simulink model "mutirotor"  (R2023a)
settings: Solver=FixedStepAuto  StartTime=0.0  StopTime=50  FixedStep=framePeriod_s  RelTol=1e-3
undefined symbols (not defined in the file): Aircraft, DiscIntNeverNeededParam, framePeriod_s, frameRate_hz, magnitude
libraries: simulink x39, slpidlib x14, dspmathops x1
(part 1 of 4)
settings Model: Creator=brian  LastModifiedBy=tuan
settings SolverCC: AlgebraicLoopSolver=TrustRegion
settings OptimizationCC: DefaultParameterBehavior=Inlined  GainParamInheritBuiltInType=on  UseFloatMulNetSlope=on  DefaultUnderspecifiedDataType=single  EnhancedBackFolding=on  BooleansAsBitfields=on  PassReuseOutputArgsAs=Individual arguments  StateBitsets=on  DataBitsets=on  ActiveStateOutputEnumStorageType=uint16  ZeroExternalMemoryAtStartup=off  ZeroInternalMemoryAtStartup=off  EfficientFloat2IntCast=on  LifeSpan=inf  DifferentSizesBufferReuse=on  OptimizationPriority=RAM  OptimizationCustomize=off  EfficientTunableParamExpr=on
settings DebuggingCC: ParameterPrecisionLossMsg=none  ParameterTunabilityLossMsg=error  UnconnectedInputMsg=warning  UnconnectedOutputMsg=warning  UnconnectedLineMsg=warning  BusObjectLabelMismatch=error  RootOutportRequireBusObject=error  NonBusSignalsTreatedAsBus=error  SFInvalidInputDataAccessInChartInitDiag=error  SFTransitionOutsideNaturalParentDiag=error  SFUnreachableExecutionPathDiag=error  SFUndirectedBroadcastEventsDiag=error
settings HardwareCC: ProdBitPerPointer=32  ProdBitPerSizeT=32  ProdBitPerPtrDiffT=32  ProdLargestAtomicInteger=Long  ProdLargestAtomicFloat=Double  ProdWordSize=32  ProdHWDeviceType=NXP->Cortex-M4  TargetLargestAtomicInteger=Long  TargetLargestAtomicFloat=Double  TargetLongLongMode=on  TargetIntDivRoundTo=Zero  TargetEndianess=LittleEndian  TargetHWDeviceType=NXP->Cortex-M4  ProdEqTarget=off
settings ModelReferenceCC: EnableRefExpFcnMdlSchedulingChecks=on  ModelReferenceNumInstancesAllowed=Single
settings SFSimCC: SimParseCustomCode=off  SimGenImportedTypeDefs=on  MATLABDynamicMemAlloc=off  SimTargetLang=C++
settings SFSimCC: SimUserIncludeDirs=|
  | ../../flight_code/include
  | ../../../ua_spaaro_extra/imu/include
  | ../../../ua_spaaro_extra/gnss/include
  | ../../../ua_spaaro_extra/pres/include
  | ../../../ua_spaaro_extra/sbus/include
  | ../../../ua_spaaro_extra/global_defs/include
settings SFSimCC: SimUserDefines=|
  | SIL
  | __FMU_R_MINI_V1__
settings RTWCC: Description=Embedded Coder  SystemTargetFile=ert.tlc  GenCodeOnly=on  TemplateMakefile=ert_default_tmf  GenerateReport=on  RTWVerbose=off  RTWUseSimCustomCode=on  Toolchain=GNU gcc/g++ | gmake (64-bit Linux)  BuildConfiguration=Specify  IncludeHyperlinkInReport=on  LaunchReport=on  TargetLang=C++  GenerateTraceInfo=on  GenerateTraceReport=on  GenerateTraceReportSl=on  GenerateTraceReportSf=on  GenerateTraceReportEml=on  GenerateCodeReplacementReport=on  DLArmComputeVersion=19.05
settings RTWCC: CustomInclude=|
  | ../../flight_code/include
  | ../../../ua_spaaro_extra/imu/include
  | ../../../ua_spaaro_extra/gnss/include
  | ../../../ua_spaaro_extra/pres/include
  | ../../../ua_spaaro_extra/sbus/include
  | ../../../ua_spaaro_extra/global_defs/include
settings RTWCC: CustomDefine=|
  | SIL
  | __FMU_R_MINI_V1__
settings CodeAppCC: ForceParamTrailComments=on  IgnoreCustomStorageClasses=off  OperatorAnnotations=on  SimulinkDataObjDesc=on  SFDataObjDesc=on  MATLABFcnDesc=on  CustomSymbolStrGlobalVar=rt$N$M  CustomSymbolStrType=$N$M  CustomSymbolStrFcn=$N$M$F  CustomSymbolStrMacro=$N$M  InsertBlockDesc=on  StateflowObjectComments=on  MATLABSourceComments=on  EnableCustomComments=on  InternalIdentifier=Classic  InlinedPrmAccess=Macros  ReqsInCode=on
settings ERTTargetCC: TargetLangStandard=C++03 (ISO)  GenerateFullHeader=off  IncludeMdlTerminateFcn=off  CombineSignalStateStructs=on  SuppressErrorStatus=on  SupportAbsoluteTime=off  CodeInterfacePackaging=C++ class  SupportNonFinite=off  SupportComplex=off  ParenthesesLevel=Standards  CastingMode=Standards  ERTHeaderFileRootName=autocode$E  ERTSourceFileRootName=autocode$E  InlinedParameterPlacement=NonHierarchical  RootIOFormat=Structure reference  ERTCustomFileTemplate=example_file_process.tlc  ERTFilePackagingFormat=Compact  PreserveExpressionOrder=on  PreserveIfCondition=on  ConvertIfToSwitch=off  EnableSignedLeftShifts=off  EnableSignedRightShifts=off  IndentSize=4

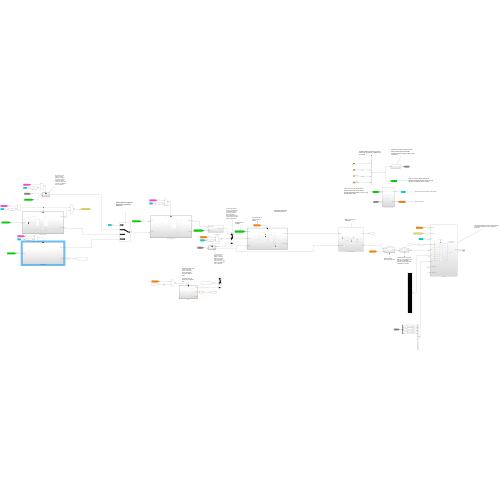
[thumbnail: Simulink's stored preview of the top-level diagram]
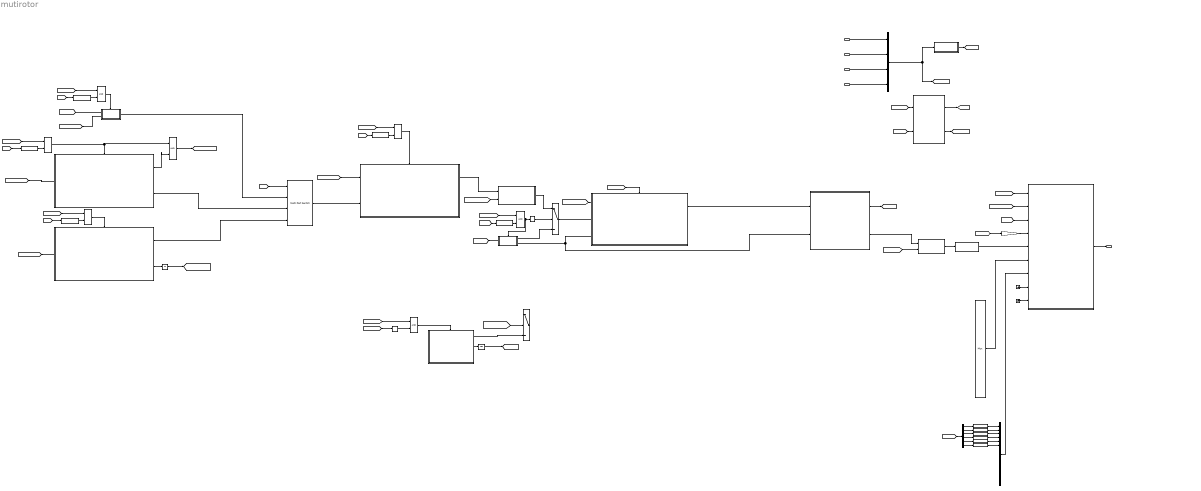
== system mutirotor ==
  note: Combine different data structures or buses into one bus for convenient of accessing
  note: Extract the inceptor channel to form some common pilot commands. Combine them to a single "cmd" bus for convenient
  note: This is a "Go To" tag. It acts like a wireless connection in the model. This is used for cleanliness of the model
  note: This is a "From" tag. It acts like a wireless connection in the model, accessing the data from the "Go To" tag with the same name
  note: This block should be used in all VMS model to format all data to the correct type for autocode.
  note: Convert motor commands from 0 to 1 into PWM value from 1100 to 1900 (or whatever range supported by the ESC or servos)
  note: System to stop motor if E-Stop is hit
  note: Motor mixing and saturation
  note: Mode signal for logging and flight_mode switching
  note: Motor arming signal
  note: ANGLE AND ANGULAR RATE CONTROLLER
  note: This ensure calc is only done when needed
  note: All data used for feedback
  note: For cascaded control scheme, controllers has a commond interface. This block switch the input of the angle control between pilot or a higher order controller based on flight mode
  note: For pilot input, the sticks can mean different command depending on flight mode. This block conver the same stick command to different state commands
  note: Autonomous Take Off mode. Just ramp motor to 70% and send it. Work well enough for MALT in cage.
      |
      | Need more testing before used anywhere else
  note: Select different input for the velocity controller interface
  note: For pilot input, the sticks can mean different command depending on flight mode. This block conver the same stick command to different state commands
  System Data : Inport  OutDataTypeStr=Bus: SysData  SampleTime=framePeriod_s  BusOutputAsStruct=on
  Sensor Data : Inport  Port=2  OutDataTypeStr=Bus: SensorData  SampleTime=framePeriod_s  BusOutputAsStruct=on
  StateEstData : Inport  Port=3  OutDataTypeStr=Bus: StateEstData  SampleTime=framePeriod_s  BusOutputAsStruct=on
  Telemetry Data : Inport  Port=4  OutDataTypeStr=Bus: TelemData  SampleTime=framePeriod_s  BusOutputAsStruct=on
  AND : Logic  IconShape=distinctive  AllPortsSameDT=off  OutDataTypeStr=boolean
  ANGLE CONTROLLER1 : Subsystem
  BODY_ACC_TO_ANGLE_CONVERSION : Subsystem
  Bus Creator1 : BusCreator  Inputs=4
  Bus Selector4 : BusSelector  OutputSignals=throttle,pitch,roll,yaw,e-stop,mode
  Cast To Single{,1..5} (6 alike) : DataTypeConversion  OutDataTypeStr=int16  SaturateOnIntegerOverflow=off  RndMeth=Floor
  Gain : Gain  Gain=100
  Ground : Ground
  Ground1 : Ground
  LAND CONTROLLER : Subsystem
  Motor Mixing Algorithm : Subsystem
  Multiport Switch : MultiPortSwitch  SaturateOnIntegerOverflow=off  InputSameDT=off
  Mux : Mux  Inputs=24
  Mux1 : Mux  Inputs=16
  NOT : Logic  Operator=NOT  IconShape=distinctive  AllPortsSameDT=off  OutDataTypeStr=boolean
  NOT1 : Logic  Operator=NOT  IconShape=distinctive  AllPortsSameDT=off  OutDataTypeStr=boolean
  POS_HOLD CONTROLLER : Subsystem
  POS_HOLD_input_conversion : Subsystem
  Stab_input_conversion : Subsystem
  Switch : Switch  Criteria=u2 > Threshold  Threshold=0.5  SaturateOnIntegerOverflow=off  InputSameDT=off
  Switch1 : Switch  Criteria=u2 > Threshold  Threshold=0.5  SaturateOnIntegerOverflow=off  InputSameDT=off
  TAKE-OFF : Subsystem
  To VMS Data1 : Subsystem
  Unit Delay : UnitDelay  SampleTime=framePeriod_s  HasFrameUpgradeWarning=on
  Unit Delay1 : UnitDelay  SampleTime=framePeriod_s  HasFrameUpgradeWarning=on
  WAYPOINT CONTROLLER : Subsystem
  cmd to raw pwm : Subsystem
  command selection : Subsystem
  compare_to_pos_hold : simulink/Logic and Bit Operations/Compare To Constant  relop=>=  const=1  OutDataTypeStr=boolean
  compare_to_stab : simulink/Logic and Bit Operations/Compare To Constant  relop===  const=0  OutDataTypeStr=boolean
  compare_to_stab1 : simulink/Logic and Bit Operations/Compare To Constant  relop===  const=1  OutDataTypeStr=boolean
  compare_to_wp : simulink/Logic and Bit Operations/Compare To Constant  relop===  const=2  OutDataTypeStr=boolean
  compare_to_wp1 : simulink/Logic and Bit Operations/Compare To Constant  relop=>=  const=3  OutDataTypeStr=boolean
  determine arm and mode selection1 : Subsystem
  emergency_stop_system : Subsystem
  motor_armed AND mode_{0..5} (6 alike) : Logic  IconShape=distinctive  AllPortsSameDT=off  OutDataTypeStr=boolean
  VmsData : Outport  OutDataTypeStr=Bus: VmsData  SampleTime=framePeriod_s  BusOutputAsStruct=on
  wires:
  To VMS Data1/1(VmsData) -> VmsData/1  "VmsData"
  [Mode] -> To VMS Data1/3(Mode in)
  [arm_state] -> To VMS Data1/1(motors_enabled)
  [throttle] -> Gain/1
  command selection/1(cmd) -> [cmd]
  Bus Creator1/1 -> command selection/1(InBus), [sys_input]
  Motor Mixing Algorithm/2(PWM) -> emergency_stop_system/1(input_signal)
  cmd to raw pwm/1(PwmCmd) -> To VMS Data1/5(PWM In)  "PwmCmd"
  emergency_stop_system/1(pwm_cmd) -> cmd to raw pwm/1(pwm_cmd)
  Mux/1 -> To VMS Data1/6(Aux)
  [arm_state] -> emergency_stop_system/2(arm)
  compare_to_stab/1 -> motor_armed AND mode_0/2
  [cmd] -> Stab_input_conversion/1(cmd)
  [sys_input] -> ANGLE CONTROLLER1/1(Sys_input)
  [arm_state] -> motor_armed AND mode_0/1
  motor_armed AND mode_0/1 -> NOT/1, Stab_input_conversion/Enable
  [Mode] -> compare_to_stab/1
  ANGLE CONTROLLER1/1(Command out) -> Motor Mixing Algorithm/1(MMA Bus)
  compare_to_pos_hold/1 -> motor_armed AND mode_1/2
  motor_armed AND mode_5/1 -> POS_HOLD_input_conversion/Enable
  [cmd] -> POS_HOLD_input_conversion/1(cmd)
  [Mode] -> compare_to_pos_hold/1
  [arm_state] -> motor_armed AND mode_1/1
  [arm_state] -> motor_armed AND mode_5/1
  [Mode] -> compare_to_stab1/1
  motor_armed AND mode_1/1 -> POS_HOLD CONTROLLER/Enable
  compare_to_stab1/1 -> motor_armed AND mode_5/2
  System Data/1 -> Bus Creator1/1  "Sys Data"
  Sensor Data/1 -> Bus Creator1/2  "Sensor Data"
  StateEstData/1 -> Bus Creator1/3  "StateEstData"
  [sys_input] -> POS_HOLD CONTROLLER/1(Sys_input)
  AND/1 -> [waypoint_reached]
  motor_armed AND mode_2/1 -> WAYPOINT CONTROLLER/Enable, AND/1
  [arm_state] -> motor_armed AND mode_2/1
  [Mode] -> compare_to_wp/1
  compare_to_wp/1 -> motor_armed AND mode_2/2
  Multiport Switch/1 -> POS_HOLD CONTROLLER/2(Cmd_input)
  [sys_input] -> WAYPOINT CONTROLLER/1(Sys_input)
  WAYPOINT CONTROLLER/1(wp_reached) -> AND/2
  [cmd] -> Bus Selector4/1
  Bus Selector4/1 -> Cast To Single/1  "<throttle>"
  Bus Selector4/2 -> Cast To Single1/1  "<pitch>"
  Bus Selector4/3 -> Cast To Single2/1  "<roll>"
  Bus Selector4/4 -> Cast To Single3/1  "<yaw>"
  Bus Selector4/5 -> Cast To Single4/1  "<e-stop>"
  Bus Selector4/6 -> Cast To Single5/1  "<mode>"
  Cast To Single/1 -> Mux1/1
  Cast To Single1/1 -> Mux1/2
  Cast To Single2/1 -> Mux1/3
  Cast To Single3/1 -> Mux1/4
  Cast To Single4/1 -> Mux1/5
  Cast To Single5/1 -> Mux1/6
  Telemetry Data/1 -> Bus Creator1/4  "Telemetry Data"
  [sys_input] -> BODY_ACC_TO_ANGLE_CONVERSION/2(SysData)
  Switch/1 -> ANGLE CONTROLLER1/2(Cmd_input)
  Motor Mixing Algorithm/1(throttle) -> [throttle]
  NOT/1 -> Switch/2
  POS_HOLD CONTROLLER/1(Command out) -> BODY_ACC_TO_ANGLE_CONVERSION/1(Outer loop command)
  BODY_ACC_TO_ANGLE_CONVERSION/1(Inner loop command) -> Switch/1
  [sys_input] -> POS_HOLD_input_conversion/2(Sys)
  POS_HOLD_input_conversion/1(angle_ctrl_input) -> Multiport Switch/2
  WAYPOINT CONTROLLER/2(wp_command) -> Multiport Switch/3
  [arm_state] -> motor_armed AND mode_3/1
  compare_to_wp1/1 -> motor_armed AND mode_3/2
  [Mode] -> compare_to_wp1/1
  motor_armed AND mode_3/1 -> LAND CONTROLLER/Enable
  [sys_input] -> LAND CONTROLLER/1(Sys_input)
  LAND CONTROLLER/2(disarm_cc) -> Unit Delay/1
  [Mode] -> Multiport Switch/1
  LAND CONTROLLER/1(land_command) -> Multiport Switch/4
  [waypoint_reached] -> To VMS Data1/2(waypoint_reached)
  Unit Delay/1 -> [LAND_DISARM]
  TAKE-OFF/2(taken_off) -> Unit Delay1/1
  Unit Delay1/1 -> [TAKEN_OFF]
  [TAKEN_OFF] -> NOT1/1
  [arm_state] -> motor_armed AND mode_4/1
  motor_armed AND mode_4/1 -> TAKE-OFF/Enable
  NOT1/1 -> motor_armed AND mode_4/2
  [TAKEN_OFF] -> Switch1/2
  [arm_state] -> ANGLE CONTROLLER1/Enable
  TAKE-OFF/1(take_off) -> Switch1/3
  Gain/1 -> To VMS Data1/4(throttle_cmd_prcnt)
  Mux1/1 -> To VMS Data1/7(SBUS in)
  Ground/1 -> To VMS Data1/8(flight_time_remaining_s)
  Ground1/1 -> To VMS Data1/9(power_remaining_prcnt)
  [sys_input] -> determine arm and mode selection1/1(sys_input)
  determine arm and mode selection1/2(arm_state) -> [arm_state]
  determine arm and mode selection1/1(mode) -> [Mode]
  [cmd] -> determine arm and mode selection1/2(Cmd)
  Stab_input_conversion/1(angle_ctrl_input) -> Switch/3
  Stab_input_conversion/2(low_throttle) -> ANGLE CONTROLLER1/3(low_thottle), Motor Mixing Algorithm/2(low_throttle_flag)

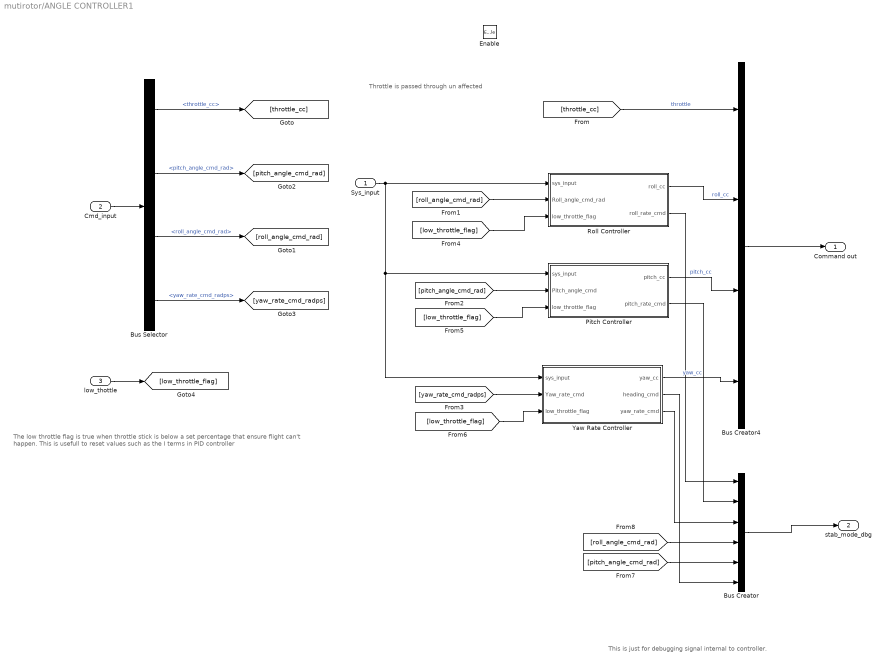
== system mutirotor/ANGLE CONTROLLER1 ==
  note: Throttle is passed through un affected
  note: The low throttle flag is true when throttle stick is below a set percentage that ensure flight can't happen. This is usefull to reset values such as the I terms in PID controller
  note: This is just for debugging signal internal to controller.
  Sys_input : Inport
  Cmd_input : Inport  Port=2
  low_thottle : Inport  Port=3
  Enable : EnablePort
  Bus Creator : BusCreator  Inputs=6
  Bus Creator4 : BusCreator  Inputs=4
  Bus Selector : BusSelector  OutputSignals=throttle_cc,pitch_angle_cmd_rad,roll_angle_cmd_rad,yaw_rate_cmd_radps
  Pitch Controller : Subsystem
  Roll Controller : Subsystem
  Yaw Rate Controller : Subsystem
  Command out : Outport
  stab_mode_dbg : Outport  Port=2
  wires:
  Bus Creator4/1 -> Command out/1
  Cmd_input/1 -> Bus Selector/1
  Yaw Rate Controller/1(yaw_cc) -> Bus Creator4/4  "yaw_cc"
  Pitch Controller/1(pitch_cc) -> Bus Creator4/3  "pitch_cc"
  Roll Controller/1(roll_cc) -> Bus Creator4/2  "roll_cc"
  Sys_input/1 -> Yaw Rate Controller/1(sys_input), Pitch Controller/1(sys_input), Roll Controller/1(sys_input)
  Bus Selector/1 -> [throttle_cc]  "<throttle_cc>"
  Bus Selector/4 -> [yaw_rate_cmd_radps]  "<yaw_rate_cmd_radps>"
  Bus Selector/2 -> [pitch_angle_cmd_rad]  "<pitch_angle_cmd_rad>"
  Bus Selector/3 -> [roll_angle_cmd_rad]  "<roll_angle_cmd_rad>"
  [throttle_cc] -> Bus Creator4/1  "throttle"
  [roll_angle_cmd_rad] -> Roll Controller/2(Roll_angle_cmd_rad)
  [pitch_angle_cmd_rad] -> Pitch Controller/2(Pitch_angle_cmd)
  [yaw_rate_cmd_radps] -> Yaw Rate Controller/2(Yaw_rate_cmd)
  low_thottle/1 -> [low_throttle_flag]
  [low_throttle_flag] -> Roll Controller/3(low_throttle_flag)
  [low_throttle_flag] -> Pitch Controller/3(low_throttle_flag)
  [low_throttle_flag] -> Yaw Rate Controller/3(low_throttle_flag)
  Roll Controller/2(roll_rate_cmd) -> Bus Creator/1
  Pitch Controller/2(pitch_rate_cmd) -> Bus Creator/2
  Bus Creator/1 -> stab_mode_dbg/1
  [roll_angle_cmd_rad] -> Bus Creator/4
  [pitch_angle_cmd_rad] -> Bus Creator/5
  Yaw Rate Controller/2(heading_cmd) -> Bus Creator/6
  Yaw Rate Controller/3(yaw_rate_cmd) -> Bus Creator/3

== system mutirotor/BODY_ACC_TO_ANGLE_CONVERSION ==
  note: The input here is the acceleration command in the earth frame in mps^2
  note: g is added to also compensate for gravity
  note: 10 deg tilt limit is pre computed
  note: Convert it to g
  note: Yaw rate command is unaffected
  note: Limit the thrust to match achivable thrust
      |
      | Prioritize vertical axis (0 lateral accel if needed)
  note: Limit max tilt of the thrust vector. Essential set a limit for tilt while ensureing the vertical accel is unchanged
  note: Conversion between thrust vector magnitude to throttle command
      |
      | The gain needs to be tunable
  note: Calculated the needed pitch and roll so that the aircraft thrust vector point in the direction of the commanded earth frame accel vector
      |
      | In this implementation, gimbal lock and inverted flight will cause problem.
      |
      | Better to implement quartenion based conversion and inner loop
  note: Construct a bus to match the inner controller interface
  Outer loop command : Inport
  SysData : Inport  Port=2
  " tilt_limiter" : MATLAB Function  TreatAsAtomicUnit=on
  Bus Creator : BusCreator  Inputs=4
  Bus Selector : BusSelector  OutputSignals=acc_x_cmd,acc_y_cmd,acc_z_cmd,yaw_rate_cmd_radps
  Bus Selector1 : BusSelector  OutputSignals=StateEstData.bfs_ins.heading_rad
  Constant : Constant  Value=Aircraft.Control.max_g_thr  OutDataTypeStr=single
  Constant1 : Constant  Value=Aircraft.Control.est_hover_thr  OutDataTypeStr=single
  Constant2 : Constant  Value=Aircraft.Control.max_g_thr  OutDataTypeStr=single
  Constant3 : Constant  Value=10  OutDataTypeStr=single
  Mux : Mux  Inputs=3
  Sum : Sum  Inputs=|+-
  calc_body_throttle : MATLAB Function  TreatAsAtomicUnit=on
  g : Constant  OutDataTypeStr=single
  normalize by g1 : Gain  Gain=1/9.81
  normalize by g2 : Gain  Gain=1/9.81
  normalize by g3 : Gain  Gain=1/9.81
  thrust_limit : MATLAB Function  TreatAsAtomicUnit=on
  tilt_command_calculation : MATLAB Function  TreatAsAtomicUnit=on
  Inner loop command : Outport
  wires:
  Constant/1 -> thrust_limit/2(max_thrust)
  Mux/1 -> thrust_limit/1(thrust_vector_raw)
  Outer loop command/1 -> Bus Selector/1
  Bus Selector/1 -> normalize by g1/1  "<acc_x_cmd>"
  Bus Selector/2 -> normalize by g2/1  "<acc_y_cmd>"
  Bus Creator/1 -> Inner loop command/1  "angle_ctrl_input"
  Bus Selector/4 -> Bus Creator/4  "<yaw_rate_cmd_radps>"
  SysData/1 -> Bus Selector1/1
  Bus Selector1/1 -> tilt_command_calculation/2(psi_rad)  "<heading_rad>"
  Bus Selector/3 -> normalize by g3/1  "<acc_z_cmd>"
  g/1 -> Sum/2
  normalize by g3/1 -> Sum/1
  normalize by g1/1 -> Mux/1
  normalize by g2/1 -> Mux/2
  Sum/1 -> Mux/3
  thrust_limit/1(limited_vector) -> " tilt_limiter"/1(thrust_vector_raw)
  tilt_command_calculation/1(phi_rad) -> Bus Creator/3  "roll_angle_cmd_rad"
  tilt_command_calculation/2(theta_rad) -> Bus Creator/2  "pitch_angle_cmd_rad"
  calc_body_throttle/1(throttle) -> Bus Creator/1  "throttle_cc"
  " tilt_limiter"/1(limited_vector) -> calc_body_throttle/1(raw_thrust_vector), tilt_command_calculation/1(thrust_vector_ned)
  Constant1/1 -> calc_body_throttle/2(hover_thr)
  Constant2/1 -> calc_body_throttle/3(max_g_thrust)
  Constant3/1 -> calc_body_throttle/4(gain)

== system mutirotor/LAND CONTROLLER ==
  note: LAND CONTROLLER IS EXPLAINED IN README
  Sys_input : Inport
  Enable : EnablePort  StatesWhenEnabling=reset  ShowOutputPort=on
  Bus Creator4 : BusCreator  Inputs=4
  Bus Selector : BusSelector  OutputSignals=Sensor Data.ext_gnss1.alt_wgs84_m
  Compare To Constant : simulink/Logic and Bit Operations/Compare To Constant  relop=<=  const=0.15  OutDataTypeStr=boolean
  Constant : Constant  Value=0  OutDataTypeStr=single
  Constant1 : Constant  Value=0  OutDataTypeStr=single
  Constant2 : Constant  Value=0  OutDataTypeStr=single
  Constant3 : Constant  Value=Aircraft.Control.v_z_max  OutDataTypeStr=single
  Enabled Subsystem : Subsystem  TreatAsAtomicUnit=on
  OR : Logic  Operator=OR  IconShape=distinctive  AllPortsSameDT=off  OutDataTypeStr=boolean
  land_command : Outport
  disarm_cc : Outport  Port=2
  wires:
  Bus Creator4/1 -> land_command/1
  Constant1/1 -> Bus Creator4/3  "ve_y_cmd_mps"
  Constant2/1 -> Bus Creator4/4  "yaw_rate_cmd_radps"
  Constant/1 -> Bus Creator4/2  "ve_x_cmd_mps"
  Constant3/1 -> Bus Creator4/1  "ve_z_cmd_mps"
  Sys_input/1 -> Bus Selector/1
  Bus Selector/1 -> Compare To Constant/1  "<alt_wgs84_m>"
  Compare To Constant/1 -> OR/1
  OR/1 -> disarm_cc/1
  Enabled Subsystem/1(LAND_MODE_TIMER) -> OR/2
  Enable/1 -> [LAND_ENABLED]
  [LAND_ENABLED] -> Enabled Subsystem/Enable

== system mutirotor/Motor Mixing Algorithm ==
  note: High level command multiply by mixing matrix
  note: Saturate minimum throttle command
  note: Extra precaution to ensure low throttle. Essentially any throttle below ~30% is no throttle at all
  note: High level commands
  MMA Bus : Inport
  low_throttle_flag : Inport  Port=2
  Bus Selector : BusSelector  OutputSignals=throttle,roll_cc,pitch_cc,yaw_cc
  Constant : Constant  OutDataTypeStr=single
  Constant1 : Constant  Value=Aircraft.Control.motor_spin_min  OutDataTypeStr=single
  Constant2 : Constant  Value=[0 0 0 0 0 0 0 0]  OutDataTypeStr=single
  Motor Mix : Constant  Value=Aircraft.Motor.mix  OutDataTypeStr=single
  Multiply : Product  Inputs=**  Multiplication=Matrix(*)  OutDataTypeStr=single
  Mux : Mux
  Reshape : Reshape  OutputDimensionality=Row vector (2-D)
  Saturation Dynamic : simulink/Discontinuities/Saturation Dynamic  OutMin=[]  OutMax=[]  OutDataTypeStr=Inherit: Same as second input  OutDataType=fixdt(1, 16)  OutScaling=2^-10  DoSatur=off
  Switch : Switch  Criteria=u2 > Threshold  SaturateOnIntegerOverflow=off  InputSameDT=off
  Transpose : Math  Operator=transpose
  throttle : Outport
  PWM : Outport  Port=2
  wires:
  Mux/1 -> Reshape/1
  Reshape/1 -> Multiply/1
  Motor Mix/1 -> Transpose/1
  MMA Bus/1 -> Bus Selector/1
  Bus Selector/1 -> Mux/1, throttle/1  "<throttle>"
  Transpose/1 -> Multiply/2
  Saturation Dynamic/1 -> PWM/1
  Constant/1 -> Saturation Dynamic/1
  Constant1/1 -> Saturation Dynamic/3
  Bus Selector/2 -> Mux/2  "<roll_cc>"
  Bus Selector/3 -> Mux/3  "<pitch_cc>"
  Bus Selector/4 -> Mux/4  "<yaw_cc>"
  Switch/1 -> Saturation Dynamic/2
  low_throttle_flag/1 -> Switch/2
  Multiply/1 -> Switch/3  "Command"
  Constant2/1 -> Switch/1

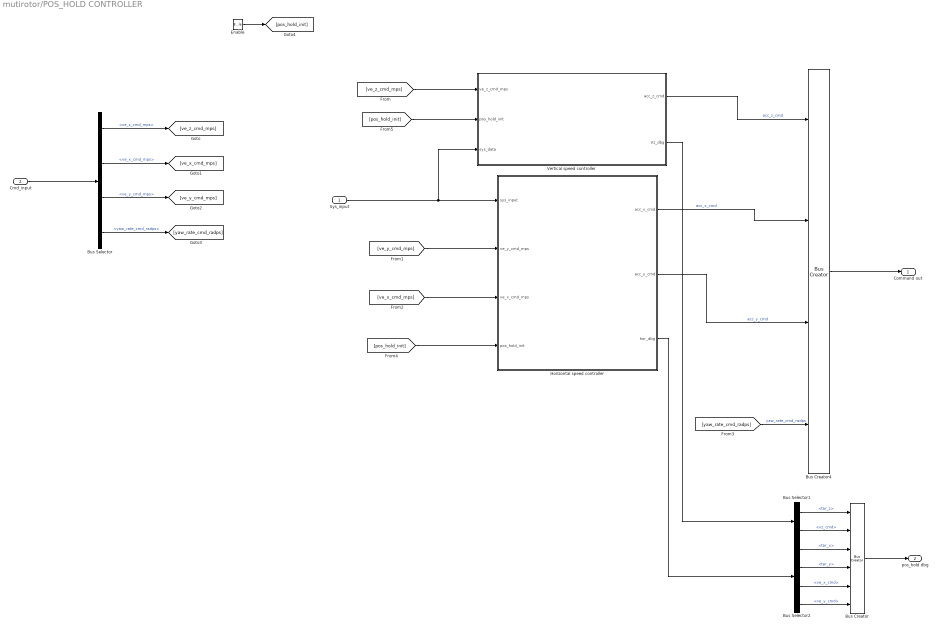
== system mutirotor/POS_HOLD CONTROLLER ==
  Sys_input : Inport
  Cmd_input : Inport  Port=2
  Enable : EnablePort  StatesWhenEnabling=reset  PropagateVarSize=During execution  ShowOutputPort=on
  Bus Creator : BusCreator  Inputs=6
  Bus Creator4 : BusCreator  Inputs=4
  Bus Selector : BusSelector  OutputSignals=ve_z_cmd_mps,ve_x_cmd_mps,ve_y_cmd_mps,yaw_rate_cmd_radps
  Bus Selector1 : BusSelector  OutputSignals=tar_z,vz_cmd
  Bus Selector2 : BusSelector  OutputSignals=tar_x,tar_y,ve_x_cmd,ve_y_cmd
  Horizontal speed controller : Subsystem
  Vertical speed controller : Subsystem
  Command out : Outport
  pos_hold dbg : Outport  Port=2
  wires:
  Bus Creator4/1 -> Command out/1
  Bus Selector/1 -> [ve_z_cmd_mps]  "<ve_z_cmd_mps>"
  Bus Selector/2 -> [ve_x_cmd_mps]  "<ve_x_cmd_mps>"
  Bus Selector/3 -> [ve_y_cmd_mps]  "<ve_y_cmd_mps>"
  Bus Selector/4 -> [yaw_rate_cmd_radps]  "<yaw_rate_cmd_radps>"
  [yaw_rate_cmd_radps] -> Bus Creator4/4  "yaw_rate_cmd_radps"
  Cmd_input/1 -> Bus Selector/1
  Enable/1 -> [pos_hold_init]
  Vertical speed controller/1(acc_z_cmd) -> Bus Creator4/1  "acc_z_cmd"
  Horizontal speed controller/1(acc_x_cmd) -> Bus Creator4/2  "acc_x_cmd"
  Horizontal speed controller/2(acc_y_cmd) -> Bus Creator4/3  "acc_y_cmd"
  [ve_y_cmd_mps] -> Horizontal speed controller/2(ve_y_cmd_mps)
  [ve_x_cmd_mps] -> Horizontal speed controller/3(ve_x_cmd_mps)
  Sys_input/1 -> Horizontal speed controller/1(sys_input), Vertical speed controller/3(sys_data)
  [pos_hold_init] -> Horizontal speed controller/4(pos_hold_init)
  [ve_z_cmd_mps] -> Vertical speed controller/1(ve_z_cmd_mps)
  [pos_hold_init] -> Vertical speed controller/2(pos_hold_init)
  Vertical speed controller/2(Vz_dbg) -> Bus Selector1/1
  Horizontal speed controller/3(hor_dbg) -> Bus Selector2/1
  Bus Selector1/1 -> Bus Creator/1  "<tar_z>"
  Bus Selector1/2 -> Bus Creator/2  "<vz_cmd>"
  Bus Selector2/1 -> Bus Creator/3  "<tar_x>"
  Bus Selector2/2 -> Bus Creator/4  "<tar_y>"
  Bus Selector2/3 -> Bus Creator/5  "<ve_x_cmd>"
  Bus Selector2/4 -> Bus Creator/6  "<ve_y_cmd>"
  Bus Creator/1 -> pos_hold dbg/1

== system mutirotor/POS_HOLD_input_conversion ==
  note: Input are yaw, pitch, roll, throttle sticj deflection
  note: Output converted to yaw rate, earth frame X, Y, and Z vel command
  note: map throttle deflection to v_z cmd directly
  note: Ensure the lateral vel commandr is constraint bby a circle (constant radius) rather than square where the corners has highest magnitude
  note: 2D rotation to convert body command to eath frame commands
  note: Yaw rate command is untouched
  cmd : Inport
  Sys : Inport  Port=2
  Enable : EnablePort
  Bus Creator : BusCreator  Inputs=4
  Bus Selector : BusSelector  OutputSignals=StateEstData.bfs_ins.heading_rad
  Bus Selector2 : BusSelector  OutputSignals=throttle,pitch,roll,yaw
  Circular constraint : MATLAB Function  TreatAsAtomicUnit=on
  Constant1 : Constant  Value=Aircraft.Control.v_hor_max  OutDataTypeStr=single
  Constant2 : Constant  Value=0.1  OutDataTypeStr=single
  Constant3 : Constant  Value=Aircraft.Control.yaw_rate_max  OutDataTypeStr=single
  Constant4 : Constant  Value=Aircraft.Control.v_hor_max  OutDataTypeStr=single
  Mux : Mux  Inputs=2
  Product : Product
  Product1 : Product
  Product2 : Product
  body_to_inertial conversion : Subsystem
  pitch_norm_deadband : Subsystem
  angle_ctrl_input : Outport
  wires:
  Bus Creator/1 -> angle_ctrl_input/1  "pos_hold_cmd"
  cmd/1 -> Bus Selector2/1
  Product/1 -> Bus Creator/4  "yaw_rate_cmd_radps"
  Bus Selector2/4 -> Product/1  "<yaw>"
  Constant1/1 -> Product1/2
  Constant4/1 -> Product2/2
  Constant3/1 -> Product/2
  Bus Selector2/1 -> pitch_norm_deadband/1(raw_sbus_in)  "<throttle>"
  pitch_norm_deadband/1(normalized_out) -> Bus Creator/1  "ve_z_cmd_mps"
  Constant2/1 -> pitch_norm_deadband/2(deadband)
  Circular constraint/1(x) -> Product1/1
  Circular constraint/2(y) -> Product2/1
  Bus Selector2/2 -> Circular constraint/1(x_in)  "<pitch>"
  Bus Selector2/3 -> Circular constraint/2(y_in)  "<roll>"
  Mux/1 -> body_to_inertial conversion/1(vb_xy)
  Product1/1 -> Mux/1  "vb_x_cmd_mps"
  Product2/1 -> Mux/2  "vb_y_cmd_mps"
  body_to_inertial conversion/1(ve_x) -> Bus Creator/2  "ve_x_cmd_mps"
  body_to_inertial conversion/2(ve_y) -> Bus Creator/3  "ve_y_cmd_mps"
  Sys/1 -> Bus Selector/1
  Bus Selector/1 -> body_to_inertial conversion/2(heading_rad)  "<heading_rad>"

== system mutirotor/Stab_input_conversion ==
  note: Ensure the tilt commandr is constraint bby a circle (constant radius) rather than square where the corners has highest magnitude
  note: low_throttle flag used by other blocks
  note: Input are yaw, pitch, roll, throttle sticj deflection
  note: Output converted to yaw rate, pitch angle, roll angle, and remapped collective throttle
  cmd : Inport
  Enable : EnablePort
  Bus Creator : BusCreator  Inputs=4
  Bus Selector2 : BusSelector  OutputSignals=throttle,pitch,roll,yaw
  Circular constraint : MATLAB Function  TreatAsAtomicUnit=on
  Compare To Constant : simulink/Logic and Bit Operations/Compare To Constant  relop=<=  const=0.03  OutDataTypeStr=boolean
  Constant : Constant  Value=Aircraft.Control.att_angle_lim  OutDataTypeStr=single
  Constant1 : Constant  Value=Aircraft.Control.att_angle_lim  OutDataTypeStr=single
  Constant2 : Constant  Value=Aircraft.Control.yaw_rate_max  OutDataTypeStr=single
  Gain : Gain  Gain=-1
  Product : Product
  Product1 : Product
  Product2 : Product
  remap from min_spin to max : Subsystem
  angle_ctrl_input : Outport
  low_throttle : Outport  Port=2
  wires:
  Product2/1 -> Bus Creator/3  "roll_angle_cmd_rad"
  Bus Selector2/2 -> Gain/1  "<pitch>"
  Bus Creator/1 -> angle_ctrl_input/1  "angle_ctrl_input"
  Product1/1 -> Bus Creator/2  "pitch_angle_cmd_rad"
  cmd/1 -> Bus Selector2/1
  Product/1 -> Bus Creator/4  "yaw_rate_cmd_radps"
  Bus Selector2/4 -> Product/1  "<yaw>"
  remap from min_spin to max/1(norm_out) -> Bus Creator/1  "throttle_cc"
  Constant/1 -> Product1/2
  Constant1/1 -> Product2/2
  Constant2/1 -> Product/2
  Bus Selector2/3 -> Circular constraint/2(y_in)  "<roll>"
  Circular constraint/2(y) -> Product2/1
  Circular constraint/1(x) -> Product1/1
  Gain/1 -> Circular constraint/1(x_in)
  Bus Selector2/1 -> Compare To Constant/1, remap from min_spin to max/1(raw_in)  "<throttle>"
  Compare To Constant/1 -> low_throttle/1

== system mutirotor/TAKE-OFF ==
  Enable : EnablePort  StatesWhenEnabling=reset
  Bus Creator : BusCreator  Inputs=4
  Compare To Constant1 : simulink/Logic and Bit Operations/Compare To Constant  relop=<=  const=0.03  OutDataTypeStr=boolean
  Compare To Constant2 : simulink/Logic and Bit Operations/Compare To Constant  relop=>=  const=0.7  OutDataTypeStr=boolean
  Constant : Constant  Value=0  OutDataTypeStr=single  SampleTime=framePeriod_s
  Constant1 : Constant  Value=0  OutDataTypeStr=single  SampleTime=framePeriod_s
  Constant2 : Constant  Value=0  OutDataTypeStr=single  SampleTime=framePeriod_s
  Constant3 : Constant  Value=0.5  OutDataTypeStr=single  SampleTime=framePeriod_s
  Constant4 : Constant  Value=framePeriod_s  OutDataTypeStr=single
  Constant5 : Constant  Value=0.5  OutDataTypeStr=single
  Delay : Delay  DelayLengthSource=Input port
      settings: InputPortMap=u0,p1
  Discrete-Time Integrator : DiscreteIntegrator  IntegratorMethod=Integration: Trapezoidal  SampleTime=framePeriod_s  OutDataTypeStr=single  LimitOutput=on  UpperSaturationLimit=0.8  LowerSaturationLimit=0  ICPrevOutput=DiscIntNeverNeededParam  ICPrevScaledInput=DiscIntNeverNeededParam
  Divide : Product  Inputs=*/
  remap from min_spin to max : Subsystem
  take_off : Outport
  taken_off : Outport  Port=2
  low_throttle : Outport  Port=3
  wires:
  Constant1/1 -> Bus Creator/3  "roll_angle_cmd_rad"
  Constant2/1 -> Bus Creator/4  "yaw_rate_cmd_radps"
  Constant/1 -> Bus Creator/2  "pitch_angle_cmd_rad"
  Bus Creator/1 -> take_off/1  "angle_ctrl_input"
  Discrete-Time Integrator/1 -> remap from min_spin to max/1(raw_in), Compare To Constant1/1  "throttle_cc"
  Compare To Constant1/1 -> low_throttle/1
  Constant3/1 -> Delay/1
  Delay/1 -> Discrete-Time Integrator/1
  Divide/1 -> Delay/2
  Constant4/1 -> Divide/2
  Constant5/1 -> Divide/1
  remap from min_spin to max/1(norm_out) -> Compare To Constant2/1, Bus Creator/1  "throttle_cc"
  Compare To Constant2/1 -> taken_off/1

== system mutirotor/To VMS Data1 ==
  note: Cast to different data types to match with definition from global_definitions.h
  note: This is the bus creator. It acts similarly to the mux in Simulink but allows user match the inputs to the an arbitrary struct. This is useful to define interfaces. Check how this bus is matching with the VMS data struct in global_definitions.h
  motors_enabled : Inport
  waypoint_reached : Inport  Port=2
  Mode in : Inport  Port=3
  throttle_cmd_prcnt : Inport  Port=4
  PWM In : Inport  Port=5
  Aux : Inport  Port=6
  SBUS in : Inport  Port=7
  flight_time_remaining_s : Inport  Port=8
  power_remaining_prcnt : Inport  Port=9
  Bus Creator : BusCreator  Inputs=9  OutDataTypeStr=Bus: VmsData  NonVirtualBus=on
      settings: InheritFromInputs=off
  Cast : DataTypeConversion  OutDataTypeStr=int8  SaturateOnIntegerOverflow=off  RndMeth=Floor
  Cast To Boolean : DataTypeConversion  OutDataTypeStr=boolean  SaturateOnIntegerOverflow=off  RndMeth=Floor
  Cast To Boolean1 : DataTypeConversion  OutDataTypeStr=boolean  SaturateOnIntegerOverflow=off  RndMeth=Floor
  Cast To Single{,1..3} (4 alike) : DataTypeConversion  OutDataTypeStr=single  SaturateOnIntegerOverflow=off  RndMeth=Floor
  Cast1 : DataTypeConversion  OutDataTypeStr=int16  SaturateOnIntegerOverflow=off  RndMeth=Floor
  Cast2 : DataTypeConversion  OutDataTypeStr=int16  SaturateOnIntegerOverflow=off  RndMeth=Floor
  VmsData : Outport
  wires:
  Bus Creator/1 -> VmsData/1
  waypoint_reached/1 -> Cast To Boolean/1  "advance_waypoint"
  motors_enabled/1 -> Cast To Boolean1/1  "motors_enabled"
  Mode in/1 -> Cast/1  "mode"
  SBUS in/1 -> Cast1/1  "sbus"
  PWM In/1 -> Cast2/1  "pwm"
  throttle_cmd_prcnt/1 -> Cast To Single1/1  "throttle_cmd_prcnt"
  Aux/1 -> Cast To Single3/1  "aux"
  Cast To Single2/1 -> Bus Creator/8  "power_remaining_prcnt"
  Cast To Single/1 -> Bus Creator/7  "flight_time_remaining_s"
  flight_time_remaining_s/1 -> Cast To Single/1  "flight_time_remaining_s"
  Cast To Boolean/1 -> Bus Creator/1  "advance_waypoint"
  Cast To Boolean1/1 -> Bus Creator/2  "motors_enabled"
  Cast/1 -> Bus Creator/3  "mode"
  Cast1/1 -> Bus Creator/4  "sbus"
  Cast2/1 -> Bus Creator/5  "pwm"
  Cast To Single1/1 -> Bus Creator/6  "throttle_cmd_prcnt"
  power_remaining_prcnt/1 -> Cast To Single2/1  "power_remaining_prcnt"
  Cast To Single3/1 -> Bus Creator/9  "aux"

== system mutirotor/WAYPOINT CONTROLLER ==
  note: Block to check if the current waypoint is reached
  note: Create signal when flight_plan is updated, wp_reached signal is true or there is an increase in waypoint index from other means
  note: Signal is used to calculate the next target position
  Sys_input : Inport
  Enable : EnablePort  StatesWhenEnabling=reset  ShowOutputPort=on
  Bus Selector1 : BusSelector  OutputSignals=Telemetry Data.waypoints_updated,Telemetry Data.current_waypoint
  Constant : Constant  OutDataTypeStr=int16
  OR : Logic  Operator=OR  Inputs=3  IconShape=distinctive  AllPortsSameDT=off  OutDataTypeStr=boolean
  Sum : Sum  Inputs=|++
  Unit Delay : UnitDelay  SampleTime=-1  HasFrameUpgradeWarning=on
  WP_NAV : Subsystem
  capture rising edge : Subsystem
  determine target : Subsystem
  wp_completion_check : Subsystem
  wp_reached : Outport
  wp_command : Outport  Port=2
  wires:
  Sys_input/1 -> Bus Selector1/1, WP_NAV/1(Sys_input), determine target/1(sys_input), wp_completion_check/2(Sys_input)
  Enable/1 -> WP_NAV/Enable
  WP_NAV/1(Command out) -> wp_command/1
  determine target/1(cur_target_pos_m) -> wp_completion_check/1(target_pos), WP_NAV/2(cur_target_pos_m)  "cur_target_pos_m"
  OR/1 -> determine target/Enable  "enable"
  Bus Selector1/1 -> OR/1  "<waypoints_updated>"
  capture rising edge/1(enable) -> OR/2
  Unit Delay/1 -> OR/3
  wp_completion_check/1(wp_reached) -> wp_reached/1, Unit Delay/1
  Constant/1 -> Sum/2
  Bus Selector1/2 -> Sum/1  "<current_waypoint>"
  Sum/1 -> capture rising edge/1(<current_waypoint>)  "cur_wp"
  determine target/2(prev_pos_m) -> WP_NAV/3(prev_pos_m)  "prev_wp"

== system mutirotor/cmd to raw pwm ==
  note: motor cmd - pwm output to actual hardware
  pwm_cmd : Inport
  Data Type Conversion : DataTypeConversion  OutDataTypeStr=int16  SaturateOnIntegerOverflow=off  RndMeth=Floor
  motor_PWM_denormalize : Subsystem
  PwmCmd : Outport
  wires:
  pwm_cmd/1 -> motor_PWM_denormalize/1(normalized_input)  "cmd"
  motor_PWM_denormalize/1(raw_output) -> Data Type Conversion/1
  Data Type Conversion/1 -> PwmCmd/1  "cnt"

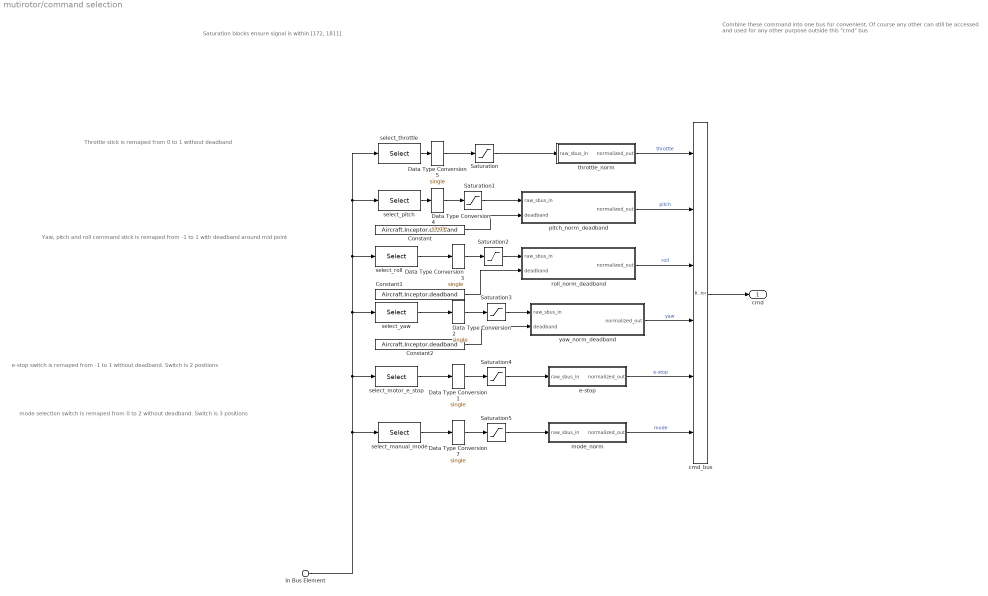
== system mutirotor/command selection ==
  note: Throttle stick is remaped from 0 to 1 without deadband
  note: Yaw, pitch and roll command stick is remaped from -1 to 1 with deadband around mid point
  note: e-stop switch is remaped from -1 to 1 without deadband. Switch is 2 positions
  note: mode selection switch is remaped from 0 to 2 without deadband. Switch is 3 positions
  note: Saturation blocks ensure signal is within [172, 1811]
  note: Combine these command into one bus for convenient. Of course any other can still be accessed and used for any other purpose outside this "cmd" bus
  In Bus Element : Inport  PortName=InBus  Element=Sensor Data.inceptor.ch
  Constant : Constant  Value=Aircraft.Inceptor.deadband  OutDataTypeStr=single
  Constant1 : Constant  Value=Aircraft.Inceptor.deadband  OutDataTypeStr=single
  Constant2 : Constant  Value=Aircraft.Inceptor.deadband  OutDataTypeStr=single
  Data Type Conversion{1..5,7} (6 alike) : DataTypeConversion  OutDataTypeStr=single  SaturateOnIntegerOverflow=off  RndMeth=Floor
  Saturation{,1..5} (6 alike) : Saturate  UpperLimit=1811  LowerLimit=172
  cmd_bus : BusCreator  Inputs=6
  e-stop : Subsystem
  mode_norm : Subsystem
  pitch_norm_deadband : Subsystem
  roll_norm_deadband : Subsystem
  select_manual_mode : Selector  IndexOptions=Index vector (dialog)  Indices=Aircraft.Inceptor.mode0  OutputSizes=1
  select_motor_e_stop : Selector  IndexOptions=Index vector (dialog)  Indices=Aircraft.Inceptor.throttle_e_stop  OutputSizes=1
  select_pitch : Selector  IndexOptions=Index vector (dialog)  Indices=Aircraft.Inceptor.pitch  OutputSizes=1
  select_roll : Selector  IndexOptions=Index vector (dialog)  Indices=Aircraft.Inceptor.roll  OutputSizes=1
  select_throttle : Selector  IndexOptions=Index vector (dialog)  Indices=Aircraft.Inceptor.throttle  OutputSizes=1
  select_yaw : Selector  IndexOptions=Index vector (dialog)  Indices=Aircraft.Inceptor.yaw  OutputSizes=1
  throttle_norm : Subsystem
  yaw_norm_deadband : Subsystem
  cmd : Outport
  wires:
  select_pitch/1 -> Data Type Conversion4/1
  select_yaw/1 -> Data Type Conversion2/1
  select_throttle/1 -> Data Type Conversion5/1
  cmd_bus/1 -> cmd/1
  Data Type Conversion5/1 -> Saturation/1
  select_roll/1 -> Data Type Conversion3/1
  Data Type Conversion1/1 -> Saturation4/1
  select_motor_e_stop/1 -> Data Type Conversion1/1
  Data Type Conversion7/1 -> Saturation5/1
  select_manual_mode/1 -> Data Type Conversion7/1
  Data Type Conversion2/1 -> Saturation3/1
  Constant2/1 -> yaw_norm_deadband/2(deadband)
  throttle_norm/1(normalized_out) -> cmd_bus/1  "throttle"
  roll_norm_deadband/1(normalized_out) -> cmd_bus/3  "roll"
  pitch_norm_deadband/1(normalized_out) -> cmd_bus/2  "pitch"
  Data Type Conversion4/1 -> Saturation1/1
  Constant/1 -> pitch_norm_deadband/2(deadband)
  Constant1/1 -> roll_norm_deadband/2(deadband)
  Data Type Conversion3/1 -> Saturation2/1
  yaw_norm_deadband/1(normalized_out) -> cmd_bus/4  "yaw"
  e-stop/1(normalized_out) -> cmd_bus/5  "e-stop"
  mode_norm/1(normalized_out) -> cmd_bus/6  "mode"
  In Bus Element/1 -> select_roll/1, select_throttle/1, select_pitch/1, select_yaw/1, select_motor_e_stop/1, select_manual_mode/1
  Saturation/1 -> throttle_norm/1(raw_sbus_in)
  Saturation1/1 -> pitch_norm_deadband/1(raw_sbus_in)
  Saturation2/1 -> roll_norm_deadband/1(raw_sbus_in)
  Saturation3/1 -> yaw_norm_deadband/1(raw_sbus_in)
  Saturation4/1 -> e-stop/1(raw_sbus_in)
  Saturation5/1 -> mode_norm/1(raw_sbus_in)

== system mutirotor/determine arm and mode selection1 ==
  note: De-bouncer ensure a signal is on continuously before register as a high or low signal
  note: This section handle how the aircraft enters autnomous LAND mode based on two OR conditions.
  note: The first condition is if telem.flight_plan.cmd[cur_wp] == 0. i.e we have reached the end of the uploaded WP list.
      |
      | Notes:
      | - Ensure that there is a flight plan uploaded because telem.flight_plan initializes to 0 so it will default to LAND there is no flight plan uploaded
      | - At the end of the mission, the aircraft lands where it is instead or RTL. This is setup for MALT for indoor cage. RTL mode need implementing
  note: The second condition is if the aircraft enters radio failsafe condition
      |
      | Notes:
      | - The aircraft will LAND as soon as radio failsafe is true
      | - Unlike Ardupilot where the aircraft RTL if in manual flight modes or continue mission if in Auto mode. This needs to be implemented
      | - This has not been tested with aircrafts other than MALT. And MALT has a special behavior compared to typical outdoor systems
  note: To emulate Ardupilot rudder arming procedure
  note: Enter LAND mode if the flag is raised via control law (LAND mode cannot be entered by the pilot).
      |
      | Otherwise, pass through manual flight mode from RC switch
  note: Allows motors to arm only if navigation filter is initialized AND manual arm_state control is to arm
  sys_input : Inport
  Cmd : Inport  Port=2
  Bus Selector1 : BusSelector  OutputSignals=mode,yaw,throttle,e-stop
  Bus Selector2 : BusSelector  OutputSignals=StateEstData.bfs_ins.initialized,Telemetry Data.flight_plan,Telemetry Data.current_waypoint,Sensor Data.inceptor
  Constant1 : Constant  Value=3  OutDataTypeStr=int8
  Land_by_failsafe : Subsystem
  Land_by_flight_plan : Subsystem
  OR1 : Logic  Operator=OR  IconShape=distinctive  AllPortsSameDT=off  OutDataTypeStr=boolean
  Switch : Switch  Criteria=u2 > Threshold  SaturateOnIntegerOverflow=off  InputSameDT=off
  e_stop de-bouncer : Subsystem
  nav_init AND motor_enable : Logic  IconShape=distinctive  AllPortsSameDT=off  OutDataTypeStr=boolean
  yaw_stick_arming : Subsystem
  mode : Outport
  arm_state : Outport  Port=2
  wires:
  sys_input/1 -> Bus Selector2/1
  Cmd/1 -> Bus Selector1/1
  Constant1/1 -> Switch/1
  [LAND_MODE] -> Switch/2
  Switch/1 -> mode/1
  Land_by_failsafe/1(radio_failsafe_enabled) -> OR1/2
  Bus Selector2/4 -> Land_by_failsafe/1(inceptor)  "<inceptor>"
  OR1/1 -> [LAND_MODE]
  Bus Selector2/1 -> nav_init AND motor_enable/1  "<initialized>"
  Bus Selector2/2 -> Land_by_flight_plan/1(<flight_plan>)  "<flight_plan>"
  Bus Selector2/3 -> Land_by_flight_plan/2(<current_waypoint>)  "<current_waypoint>"
  Land_by_flight_plan/1(is_land_cmd) -> OR1/1
  nav_init AND motor_enable/1 -> arm_state/1
  Bus Selector1/4 -> e_stop de-bouncer/1(<e_stop>)  "<e-stop>"
  Bus Selector1/1 -> Switch/3  "<mode>"
  Bus Selector1/2 -> yaw_stick_arming/1(<yaw>)  "<yaw>"
  Bus Selector1/3 -> yaw_stick_arming/2(<throttle>)  "<throttle>"
  e_stop de-bouncer/1(e_stop_filtered) -> yaw_stick_arming/3(e_stop)
  yaw_stick_arming/1(arm_state) -> nav_init AND motor_enable/2

== system mutirotor/emergency_stop_system ==
  input_signal : Inport
  arm : Inport  Port=2
  Constant : Constant  Value=[0,0,0,0,0,0,0,0]  OutDataTypeStr=single
  emergency_switch : Switch  Criteria=u2 > Threshold  Threshold=0.5  SaturateOnIntegerOverflow=off  InputSameDT=off
  pwm_cmd : Outport
  wires:
  emergency_switch/1 -> pwm_cmd/1
  arm/1 -> emergency_switch/2
  input_signal/1 -> emergency_switch/1
  Constant/1 -> emergency_switch/3
